simulink model "path_estimation"  (R2023b)
settings: Solver=FixedStepAuto  StartTime=0.0  StopTime=inf  RelTol=1e-3  EnableMultiTasking=on
undefined symbols (not defined in the file): hw
libraries: matrix_library x42, dspadpt3 x20, raspberrypiAVlib x2, audiosources x1
settings Model: ExtModeTrigDuration=2  Creator=mykni  LastModifiedBy=aaron
settings SolverCC: PositivePriorityOrder=on
settings OptimizationCC: EnhancedBackFolding=on  PassReuseOutputArgsAs=Individual arguments  ZeroExternalMemoryAtStartup=off  ZeroInternalMemoryAtStartup=off  MaxStackSize=64  OptimizeBlockOrder=speed  DifferentSizesBufferReuse=on  OptimizationCustomize=off  EfficientTunableParamExpr=on
settings DebuggingCC: ParameterTunabilityLossMsg=error
settings HardwareCC: ProdBitPerPointer=32  ProdBitPerSizeT=32  ProdBitPerPtrDiffT=32  ProdLargestAtomicInteger=Long  ProdLargestAtomicFloat=Double  ProdWordSize=32  ProdLongLongMode=on  ProdHWDeviceType=ARM Compatible->ARM Cortex  UseEmbeddedCoderFeatures=off  UseSimulinkCoderFeatures=off
settings RTWCC: Description=Embedded Coder  SystemTargetFile=ert.tlc  HardwareBoard=Raspberry Pi  TLCOptions="-aInlineSetEventsForThisBaseRateFcn=TLC_FALSE -aSuppressMultiTaskScheduler=TLC_FALSE  -aRateBasedStepFcn=0"  TemplateMakefile=ert_default_tmf  Toolchain=GNU GCC Embedded Linux  BuildConfiguration=Faster Runs
settings CodeAppCC: ForceParamTrailComments=on  IgnoreCustomStorageClasses=off  OperatorAnnotations=on  SimulinkDataObjDesc=on  SFDataObjDesc=on  InsertBlockDesc=on
settings ERTTargetCC: SupportNonInlinedSFcns=on  SupportVariableSizeSignals=on  ExtModeTransport=2  ExtModeStaticAlloc=on  ExtModeMexFile=ext_xcp  ExtModeIntrfLevel=Level2 - Open

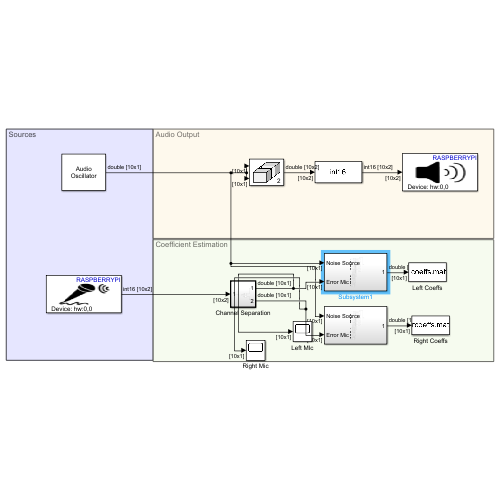
[thumbnail: Simulink's stored preview of the top-level diagram]
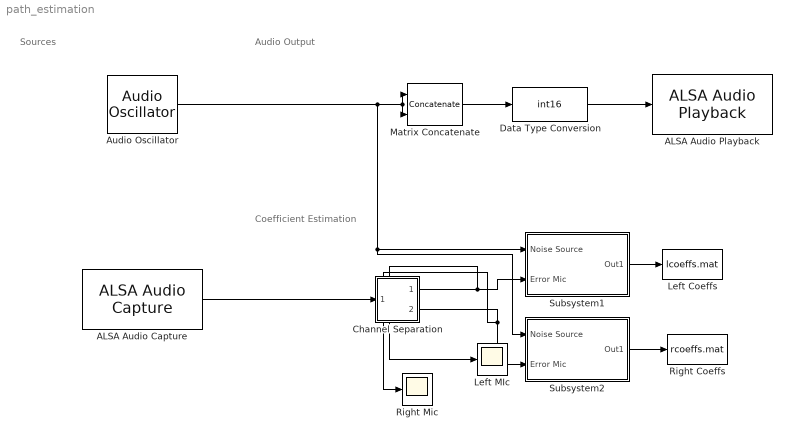
== system path_estimation ==
  note: Audio Output
  note: Coefficient Estimation
  note: Sources
  ALSA Audio Capture : raspberrypiAVlib/ALSA Audio Capture  deviceStr=hw:0,0  DataBitDepth=16-bit integer  numberOfChannels=2  sampleRateEnum=44100  frameSize=10  QueueDuration=0.5  blockPlatform=LINUX
  ALSA Audio Playback : raspberrypiAVlib/ALSA Audio Playback  deviceStr=hw:0,0  sampleRateEnum=44100  queueDuration=0.5  blockPlatform=LINUX
  Audio Oscillator : audiosources/Audio Oscillator  FrequencyPort=off  Frequency=300  AmplitudePort=off  Amplitude=3*10^4  DCOffsetPort=off  PhaseOffset=0  DCOffset=0  WidthPort=off  Width=1  DutyCyclePort=off  DutyCycle=0.5  SampsPerFrame=10  Fs=44100  OutputDataType=double  SimulateUsing=Code generation
      settings: SignalType=sine
  Channel Separation : Subsystem  TreatAsAtomicUnit=on
  Data Type Conversion : DataTypeConversion  OutDataTypeStr=int16  SaturateOnIntegerOverflow=off  RndMeth=Floor
  Left Coeffs : ToFile  Filename=lcoeffs.mat
  Left MIc : Scope
  Matrix Concatenate : Concatenate  Mode=Multidimensional array  ConcatenateDimension=2
  Right Coeffs : ToFile  Filename=rcoeffs.mat
  Right Mic : Scope
  Subsystem1 : Subsystem
  Subsystem2 : Subsystem
  wires:
  Matrix Concatenate/1 -> Data Type Conversion/1
  Audio Oscillator/1 -> Matrix Concatenate/2, Matrix Concatenate/1, Subsystem2/1(Noise Source), Subsystem1/1(Noise Source)
  ALSA Audio Capture/1 -> Channel Separation/1(In1)
  Channel Separation/1(Out1) -> Left MIc/1, Subsystem1/2(Error Mic)
  Channel Separation/2(Out2) -> Right Mic/1, Subsystem2/2(Error Mic)
  Data Type Conversion/1 -> ALSA Audio Playback/1
  Subsystem1/1(Out1) -> Left Coeffs/1
  Subsystem2/1(Out1) -> Right Coeffs/1

== system path_estimation/Channel Separation ==
  In1 : Inport
  Cast To Double : DataTypeConversion  OutDataTypeStr=double  SaturateOnIntegerOverflow=off  RndMeth=Floor
  Submatrix : matrix_library/Submatrix  RowSpan=All rows  RowStartMode=First  RowStartIndex=1  RowEndMode=Last  RowEndIndex=1  ColSpan=One column  ColStartMode=First  ColStartIndex=1  ColEndMode=Last  ColEndIndex=1
  Submatrix1 : matrix_library/Submatrix  RowSpan=All rows  RowStartMode=First  RowStartIndex=1  RowEndMode=Last  RowEndIndex=1  ColSpan=One column  ColStartMode=Last  ColStartIndex=1  ColEndMode=Last  ColEndIndex=1
  Out1 : Outport
  Out2 : Outport  Port=2
  wires:
  Submatrix1/1 -> Out2/1
  Submatrix/1 -> Out1/1
  Cast To Double/1 -> Submatrix1/1, Submatrix/1
  In1/1 -> Cast To Double/1

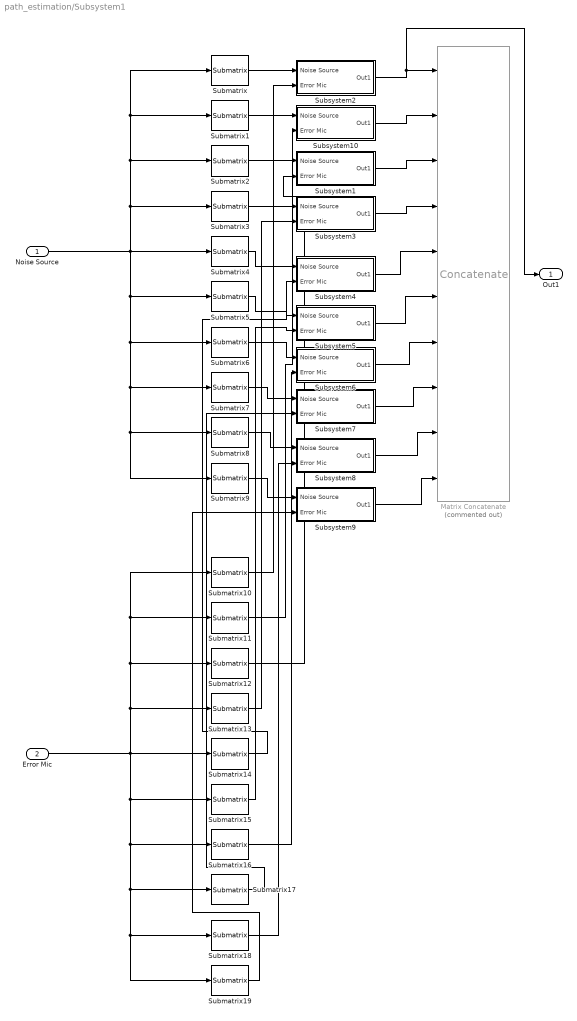
== system path_estimation/Subsystem1 ==
  Noise Source : Inport
  Error Mic : Inport  Port=2
  Matrix Concatenate : Concatenate  Commented=on  NumInputs=10  Mode=Multidimensional array
  Submatrix : matrix_library/Submatrix  RowSpan=One row  RowStartMode=Index  RowStartIndex=1  RowEndMode=Last  RowEndIndex=1  ColSpan=One column  ColStartMode=First  ColStartIndex=1  ColEndMode=Last  ColEndIndex=1
  Submatrix1 : matrix_library/Submatrix  RowSpan=One row  RowStartMode=Index  RowStartIndex=2  RowEndMode=Last  RowEndIndex=1  ColSpan=One column  ColStartMode=First  ColStartIndex=1  ColEndMode=Last  ColEndIndex=1
  Submatrix10 : matrix_library/Submatrix  RowSpan=One row  RowStartMode=Index  RowStartIndex=1  RowEndMode=Last  RowEndIndex=1  ColSpan=One column  ColStartMode=First  ColStartIndex=1  ColEndMode=Last  ColEndIndex=1
  Submatrix11 : matrix_library/Submatrix  RowSpan=One row  RowStartMode=Index  RowStartIndex=2  RowEndMode=Last  RowEndIndex=1  ColSpan=One column  ColStartMode=First  ColStartIndex=1  ColEndMode=Last  ColEndIndex=1
  Submatrix12 : matrix_library/Submatrix  RowSpan=One row  RowStartMode=Index  RowStartIndex=3  RowEndMode=Last  RowEndIndex=1  ColSpan=One column  ColStartMode=First  ColStartIndex=1  ColEndMode=Last  ColEndIndex=1
  Submatrix13 : matrix_library/Submatrix  RowSpan=One row  RowStartMode=Index  RowStartIndex=4  RowEndMode=Last  RowEndIndex=1  ColSpan=One column  ColStartMode=First  ColStartIndex=1  ColEndMode=Last  ColEndIndex=1
  Submatrix14 : matrix_library/Submatrix  RowSpan=One row  RowStartMode=Index  RowStartIndex=5  RowEndMode=Last  RowEndIndex=1  ColSpan=One column  ColStartMode=First  ColStartIndex=1  ColEndMode=Last  ColEndIndex=1
  Submatrix15 : matrix_library/Submatrix  RowSpan=One row  RowStartMode=Index  RowStartIndex=6  RowEndMode=Last  RowEndIndex=1  ColSpan=One column  ColStartMode=First  ColStartIndex=1  ColEndMode=Last  ColEndIndex=1
  Submatrix16 : matrix_library/Submatrix  RowSpan=One row  RowStartMode=Index  RowStartIndex=7  RowEndMode=Last  RowEndIndex=1  ColSpan=One column  ColStartMode=First  ColStartIndex=1  ColEndMode=Last  ColEndIndex=1
  Submatrix17 : matrix_library/Submatrix  RowSpan=One row  RowStartMode=Index  RowStartIndex=8  RowEndMode=Last  RowEndIndex=1  ColSpan=One column  ColStartMode=First  ColStartIndex=1  ColEndMode=Last  ColEndIndex=1
  Submatrix18 : matrix_library/Submatrix  RowSpan=One row  RowStartMode=Index  RowStartIndex=9  RowEndMode=Last  RowEndIndex=1  ColSpan=One column  ColStartMode=First  ColStartIndex=1  ColEndMode=Last  ColEndIndex=1
  Submatrix19 : matrix_library/Submatrix  RowSpan=One row  RowStartMode=Index  RowStartIndex=10  RowEndMode=Last  RowEndIndex=1  ColSpan=One column  ColStartMode=First  ColStartIndex=1  ColEndMode=Last  ColEndIndex=1
  Submatrix2 : matrix_library/Submatrix  RowSpan=One row  RowStartMode=Index  RowStartIndex=3  RowEndMode=Last  RowEndIndex=1  ColSpan=One column  ColStartMode=First  ColStartIndex=1  ColEndMode=Last  ColEndIndex=1
  Submatrix3 : matrix_library/Submatrix  RowSpan=One row  RowStartMode=Index  RowStartIndex=4  RowEndMode=Last  RowEndIndex=1  ColSpan=One column  ColStartMode=First  ColStartIndex=1  ColEndMode=Last  ColEndIndex=1
  Submatrix4 : matrix_library/Submatrix  RowSpan=One row  RowStartMode=Index  RowStartIndex=5  RowEndMode=Last  RowEndIndex=1  ColSpan=One column  ColStartMode=First  ColStartIndex=1  ColEndMode=Last  ColEndIndex=1
  Submatrix5 : matrix_library/Submatrix  RowSpan=One row  RowStartMode=Index  RowStartIndex=6  RowEndMode=Last  RowEndIndex=1  ColSpan=One column  ColStartMode=First  ColStartIndex=1  ColEndMode=Last  ColEndIndex=1
  Submatrix6 : matrix_library/Submatrix  RowSpan=One row  RowStartMode=Index  RowStartIndex=7  RowEndMode=Last  RowEndIndex=1  ColSpan=One column  ColStartMode=First  ColStartIndex=1  ColEndMode=Last  ColEndIndex=1
  Submatrix7 : matrix_library/Submatrix  RowSpan=One row  RowStartMode=Index  RowStartIndex=8  RowEndMode=Last  RowEndIndex=1  ColSpan=One column  ColStartMode=First  ColStartIndex=1  ColEndMode=Last  ColEndIndex=1
  Submatrix8 : matrix_library/Submatrix  RowSpan=One row  RowStartMode=Index  RowStartIndex=9  RowEndMode=Last  RowEndIndex=1  ColSpan=One column  ColStartMode=First  ColStartIndex=1  ColEndMode=Last  ColEndIndex=1
  Submatrix9 : matrix_library/Submatrix  RowSpan=One row  RowStartMode=Index  RowStartIndex=10  RowEndMode=Last  RowEndIndex=1  ColSpan=One column  ColStartMode=First  ColStartIndex=1  ColEndMode=Last  ColEndIndex=1
  Subsystem1 : Subsystem
  Subsystem10 : Subsystem
  Subsystem2 : Subsystem
  Subsystem3 : Subsystem
  Subsystem4 : Subsystem
  Subsystem5 : Subsystem
  Subsystem6 : Subsystem
  Subsystem7 : Subsystem
  Subsystem8 : Subsystem
  Subsystem9 : Subsystem
  Out1 : Outport
  wires:
  Noise Source/1 -> Submatrix9/1, Submatrix8/1, Submatrix7/1, Submatrix6/1, Submatrix5/1, Submatrix/1, Submatrix1/1, Submatrix2/1, Submatrix3/1, Submatrix4/1
  Submatrix/1 -> Subsystem2/1(Noise Source)
  Error Mic/1 -> Submatrix19/1, Submatrix18/1, Submatrix17/1, Submatrix16/1, Submatrix15/1, Submatrix10/1, Submatrix11/1, Submatrix12/1, Submatrix13/1, Submatrix14/1
  Submatrix10/1 -> Subsystem2/2(Error Mic)
  Submatrix1/1 -> Subsystem10/1(Noise Source)
  Submatrix11/1 -> Subsystem10/2(Error Mic)
  Submatrix2/1 -> Subsystem1/1(Noise Source)
  Submatrix12/1 -> Subsystem1/2(Error Mic)
  Submatrix3/1 -> Subsystem3/1(Noise Source)
  Submatrix13/1 -> Subsystem3/2(Error Mic)
  Submatrix4/1 -> Subsystem4/1(Noise Source)
  Submatrix14/1 -> Subsystem4/2(Error Mic)
  Subsystem4/1(Out1) -> Matrix Concatenate/5
  Submatrix5/1 -> Subsystem5/1(Noise Source)
  Submatrix15/1 -> Subsystem5/2(Error Mic)
  Subsystem5/1(Out1) -> Matrix Concatenate/6
  Submatrix6/1 -> Subsystem6/1(Noise Source)
  Submatrix16/1 -> Subsystem6/2(Error Mic)
  Submatrix17/1 -> Subsystem7/2(Error Mic)
  Submatrix7/1 -> Subsystem7/1(Noise Source)
  Subsystem7/1(Out1) -> Matrix Concatenate/8
  Subsystem6/1(Out1) -> Matrix Concatenate/7
  Subsystem8/1(Out1) -> Matrix Concatenate/9
  Subsystem9/1(Out1) -> Matrix Concatenate/10
  Submatrix8/1 -> Subsystem8/1(Noise Source)
  Submatrix9/1 -> Subsystem9/1(Noise Source)
  Submatrix18/1 -> Subsystem8/2(Error Mic)
  Submatrix19/1 -> Subsystem9/2(Error Mic)
  Subsystem3/1(Out1) -> Matrix Concatenate/4
  Subsystem2/1(Out1) -> Out1/1, Matrix Concatenate/1
  Subsystem10/1(Out1) -> Matrix Concatenate/2
  Subsystem1/1(Out1) -> Matrix Concatenate/3

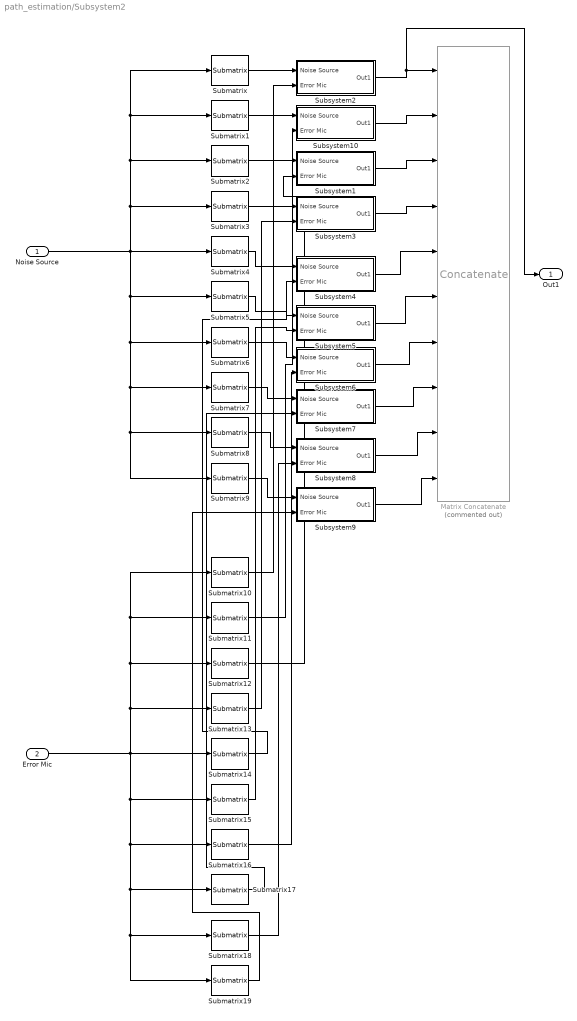
== system path_estimation/Subsystem2 ==
  Noise Source : Inport
  Error Mic : Inport  Port=2
  Matrix Concatenate : Concatenate  Commented=on  NumInputs=10  Mode=Multidimensional array
  Submatrix : matrix_library/Submatrix  RowSpan=One row  RowStartMode=Index  RowStartIndex=1  RowEndMode=Last  RowEndIndex=1  ColSpan=One column  ColStartMode=First  ColStartIndex=1  ColEndMode=Last  ColEndIndex=1
  Submatrix1 : matrix_library/Submatrix  RowSpan=One row  RowStartMode=Index  RowStartIndex=2  RowEndMode=Last  RowEndIndex=1  ColSpan=One column  ColStartMode=First  ColStartIndex=1  ColEndMode=Last  ColEndIndex=1
  Submatrix10 : matrix_library/Submatrix  RowSpan=One row  RowStartMode=Index  RowStartIndex=1  RowEndMode=Last  RowEndIndex=1  ColSpan=One column  ColStartMode=First  ColStartIndex=1  ColEndMode=Last  ColEndIndex=1
  Submatrix11 : matrix_library/Submatrix  RowSpan=One row  RowStartMode=Index  RowStartIndex=2  RowEndMode=Last  RowEndIndex=1  ColSpan=One column  ColStartMode=First  ColStartIndex=1  ColEndMode=Last  ColEndIndex=1
  Submatrix12 : matrix_library/Submatrix  RowSpan=One row  RowStartMode=Index  RowStartIndex=3  RowEndMode=Last  RowEndIndex=1  ColSpan=One column  ColStartMode=First  ColStartIndex=1  ColEndMode=Last  ColEndIndex=1
  Submatrix13 : matrix_library/Submatrix  RowSpan=One row  RowStartMode=Index  RowStartIndex=4  RowEndMode=Last  RowEndIndex=1  ColSpan=One column  ColStartMode=First  ColStartIndex=1  ColEndMode=Last  ColEndIndex=1
  Submatrix14 : matrix_library/Submatrix  RowSpan=One row  RowStartMode=Index  RowStartIndex=5  RowEndMode=Last  RowEndIndex=1  ColSpan=One column  ColStartMode=First  ColStartIndex=1  ColEndMode=Last  ColEndIndex=1
  Submatrix15 : matrix_library/Submatrix  RowSpan=One row  RowStartMode=Index  RowStartIndex=6  RowEndMode=Last  RowEndIndex=1  ColSpan=One column  ColStartMode=First  ColStartIndex=1  ColEndMode=Last  ColEndIndex=1
  Submatrix16 : matrix_library/Submatrix  RowSpan=One row  RowStartMode=Index  RowStartIndex=7  RowEndMode=Last  RowEndIndex=1  ColSpan=One column  ColStartMode=First  ColStartIndex=1  ColEndMode=Last  ColEndIndex=1
  Submatrix17 : matrix_library/Submatrix  RowSpan=One row  RowStartMode=Index  RowStartIndex=8  RowEndMode=Last  RowEndIndex=1  ColSpan=One column  ColStartMode=First  ColStartIndex=1  ColEndMode=Last  ColEndIndex=1
  Submatrix18 : matrix_library/Submatrix  RowSpan=One row  RowStartMode=Index  RowStartIndex=9  RowEndMode=Last  RowEndIndex=1  ColSpan=One column  ColStartMode=First  ColStartIndex=1  ColEndMode=Last  ColEndIndex=1
  Submatrix19 : matrix_library/Submatrix  RowSpan=One row  RowStartMode=Index  RowStartIndex=10  RowEndMode=Last  RowEndIndex=1  ColSpan=One column  ColStartMode=First  ColStartIndex=1  ColEndMode=Last  ColEndIndex=1
  Submatrix2 : matrix_library/Submatrix  RowSpan=One row  RowStartMode=Index  RowStartIndex=3  RowEndMode=Last  RowEndIndex=1  ColSpan=One column  ColStartMode=First  ColStartIndex=1  ColEndMode=Last  ColEndIndex=1
  Submatrix3 : matrix_library/Submatrix  RowSpan=One row  RowStartMode=Index  RowStartIndex=4  RowEndMode=Last  RowEndIndex=1  ColSpan=One column  ColStartMode=First  ColStartIndex=1  ColEndMode=Last  ColEndIndex=1
  Submatrix4 : matrix_library/Submatrix  RowSpan=One row  RowStartMode=Index  RowStartIndex=5  RowEndMode=Last  RowEndIndex=1  ColSpan=One column  ColStartMode=First  ColStartIndex=1  ColEndMode=Last  ColEndIndex=1
  Submatrix5 : matrix_library/Submatrix  RowSpan=One row  RowStartMode=Index  RowStartIndex=6  RowEndMode=Last  RowEndIndex=1  ColSpan=One column  ColStartMode=First  ColStartIndex=1  ColEndMode=Last  ColEndIndex=1
  Submatrix6 : matrix_library/Submatrix  RowSpan=One row  RowStartMode=Index  RowStartIndex=7  RowEndMode=Last  RowEndIndex=1  ColSpan=One column  ColStartMode=First  ColStartIndex=1  ColEndMode=Last  ColEndIndex=1
  Submatrix7 : matrix_library/Submatrix  RowSpan=One row  RowStartMode=Index  RowStartIndex=8  RowEndMode=Last  RowEndIndex=1  ColSpan=One column  ColStartMode=First  ColStartIndex=1  ColEndMode=Last  ColEndIndex=1
  Submatrix8 : matrix_library/Submatrix  RowSpan=One row  RowStartMode=Index  RowStartIndex=9  RowEndMode=Last  RowEndIndex=1  ColSpan=One column  ColStartMode=First  ColStartIndex=1  ColEndMode=Last  ColEndIndex=1
  Submatrix9 : matrix_library/Submatrix  RowSpan=One row  RowStartMode=Index  RowStartIndex=10  RowEndMode=Last  RowEndIndex=1  ColSpan=One column  ColStartMode=First  ColStartIndex=1  ColEndMode=Last  ColEndIndex=1
  Subsystem1 : Subsystem
  Subsystem10 : Subsystem
  Subsystem2 : Subsystem
  Subsystem3 : Subsystem
  Subsystem4 : Subsystem
  Subsystem5 : Subsystem
  Subsystem6 : Subsystem
  Subsystem7 : Subsystem
  Subsystem8 : Subsystem
  Subsystem9 : Subsystem
  Out1 : Outport
  wires:
  Noise Source/1 -> Submatrix9/1, Submatrix8/1, Submatrix7/1, Submatrix6/1, Submatrix5/1, Submatrix/1, Submatrix1/1, Submatrix2/1, Submatrix3/1, Submatrix4/1
  Submatrix/1 -> Subsystem2/1(Noise Source)
  Error Mic/1 -> Submatrix19/1, Submatrix18/1, Submatrix17/1, Submatrix16/1, Submatrix15/1, Submatrix10/1, Submatrix11/1, Submatrix12/1, Submatrix13/1, Submatrix14/1
  Submatrix10/1 -> Subsystem2/2(Error Mic)
  Submatrix1/1 -> Subsystem10/1(Noise Source)
  Submatrix11/1 -> Subsystem10/2(Error Mic)
  Submatrix2/1 -> Subsystem1/1(Noise Source)
  Submatrix12/1 -> Subsystem1/2(Error Mic)
  Submatrix3/1 -> Subsystem3/1(Noise Source)
  Submatrix13/1 -> Subsystem3/2(Error Mic)
  Submatrix4/1 -> Subsystem4/1(Noise Source)
  Submatrix14/1 -> Subsystem4/2(Error Mic)
  Subsystem4/1(Out1) -> Matrix Concatenate/5
  Submatrix5/1 -> Subsystem5/1(Noise Source)
  Submatrix15/1 -> Subsystem5/2(Error Mic)
  Subsystem5/1(Out1) -> Matrix Concatenate/6
  Submatrix6/1 -> Subsystem6/1(Noise Source)
  Submatrix16/1 -> Subsystem6/2(Error Mic)
  Submatrix17/1 -> Subsystem7/2(Error Mic)
  Submatrix7/1 -> Subsystem7/1(Noise Source)
  Subsystem7/1(Out1) -> Matrix Concatenate/8
  Subsystem6/1(Out1) -> Matrix Concatenate/7
  Subsystem8/1(Out1) -> Matrix Concatenate/9
  Subsystem9/1(Out1) -> Matrix Concatenate/10
  Submatrix8/1 -> Subsystem8/1(Noise Source)
  Submatrix9/1 -> Subsystem9/1(Noise Source)
  Submatrix18/1 -> Subsystem8/2(Error Mic)
  Submatrix19/1 -> Subsystem9/2(Error Mic)
  Subsystem3/1(Out1) -> Matrix Concatenate/4
  Subsystem2/1(Out1) -> Out1/1, Matrix Concatenate/1
  Subsystem10/1(Out1) -> Matrix Concatenate/2
  Subsystem1/1(Out1) -> Matrix Concatenate/3

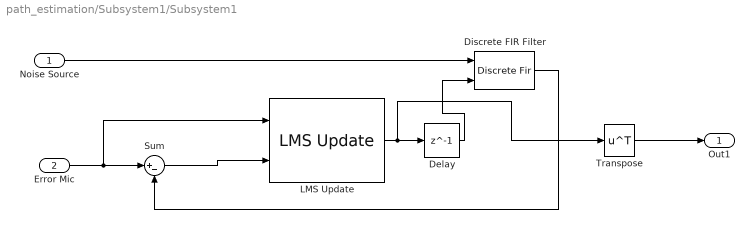
== system path_estimation/Subsystem1/Subsystem1 ==
  Noise Source : Inport
  Error Mic : Inport  Port=2
  Delay : Delay  DelayLength=1  InitialCondition=0
  Discrete FIR Filter : DiscreteFir  CoefSource=Input port
      settings: InputPortMap=u0,u1
  LMS Update : dspadpt3/LMS Update  Method=LMS  Length=10  NumFilters=1  StepSizeSource=Property  StepSize=0.1  LeakageFactor=1.0  InitialConditions=0  AdaptiveFilterMode=Tapped delay-line FIR filter  EnableAdaptInput=off  EnableResetInput=off  SimulateUsing=Code generation
  Sum : Sum  Inputs=|+-
  Transpose : Math  Operator=transpose
  Out1 : Outport
  wires:
  LMS Update/1 -> Transpose/1, Delay/1
  Delay/1 -> Discrete FIR Filter/2
  Noise Source/1 -> Discrete FIR Filter/1
  Error Mic/1 -> LMS Update/1, Sum/1
  Sum/1 -> LMS Update/2
  Discrete FIR Filter/1 -> Sum/2
  Transpose/1 -> Out1/1

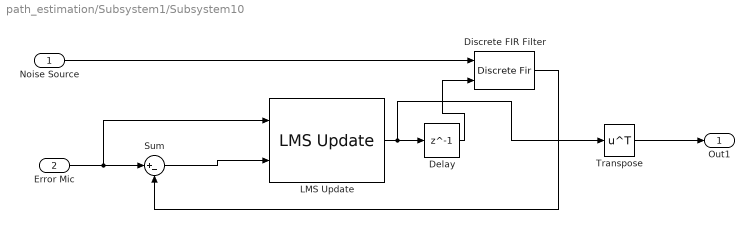
== system path_estimation/Subsystem1/Subsystem10 ==
  Noise Source : Inport
  Error Mic : Inport  Port=2
  Delay : Delay  DelayLength=1  InitialCondition=0
  Discrete FIR Filter : DiscreteFir  CoefSource=Input port
      settings: InputPortMap=u0,u1
  LMS Update : dspadpt3/LMS Update  Method=LMS  Length=10  NumFilters=1  StepSizeSource=Property  StepSize=0.1  LeakageFactor=1.0  InitialConditions=0  AdaptiveFilterMode=Tapped delay-line FIR filter  EnableAdaptInput=off  EnableResetInput=off  SimulateUsing=Code generation
  Sum : Sum  Inputs=|+-
  Transpose : Math  Operator=transpose
  Out1 : Outport
  wires:
  LMS Update/1 -> Transpose/1, Delay/1
  Delay/1 -> Discrete FIR Filter/2
  Noise Source/1 -> Discrete FIR Filter/1
  Error Mic/1 -> LMS Update/1, Sum/1
  Sum/1 -> LMS Update/2
  Discrete FIR Filter/1 -> Sum/2
  Transpose/1 -> Out1/1

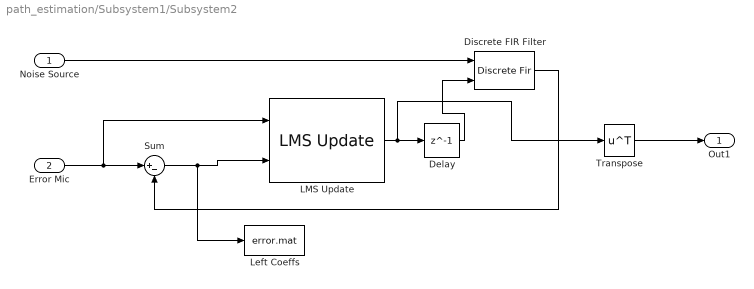
== system path_estimation/Subsystem1/Subsystem2 ==
  Noise Source : Inport
  Error Mic : Inport  Port=2
  Delay : Delay  DelayLength=1  InitialCondition=0
  Discrete FIR Filter : DiscreteFir  CoefSource=Input port
      settings: InputPortMap=u0,u1
  LMS Update : dspadpt3/LMS Update  Method=LMS  Length=10  NumFilters=1  StepSizeSource=Property  StepSize=0.1  LeakageFactor=1.0  InitialConditions=0  AdaptiveFilterMode=Tapped delay-line FIR filter  EnableAdaptInput=off  EnableResetInput=off  SimulateUsing=Code generation
  Left Coeffs : ToFile  Filename=error.mat
  Sum : Sum  Inputs=|+-
  Transpose : Math  Operator=transpose
  Out1 : Outport
  wires:
  LMS Update/1 -> Transpose/1, Delay/1
  Delay/1 -> Discrete FIR Filter/2
  Noise Source/1 -> Discrete FIR Filter/1
  Error Mic/1 -> LMS Update/1, Sum/1
  Sum/1 -> Left Coeffs/1, LMS Update/2
  Discrete FIR Filter/1 -> Sum/2
  Transpose/1 -> Out1/1

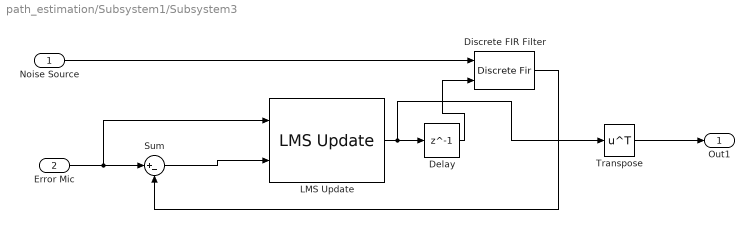
== system path_estimation/Subsystem1/Subsystem3 ==
  Noise Source : Inport
  Error Mic : Inport  Port=2
  Delay : Delay  DelayLength=1  InitialCondition=0
  Discrete FIR Filter : DiscreteFir  CoefSource=Input port
      settings: InputPortMap=u0,u1
  LMS Update : dspadpt3/LMS Update  Method=LMS  Length=10  NumFilters=1  StepSizeSource=Property  StepSize=0.1  LeakageFactor=1.0  InitialConditions=0  AdaptiveFilterMode=Tapped delay-line FIR filter  EnableAdaptInput=off  EnableResetInput=off  SimulateUsing=Code generation
  Sum : Sum  Inputs=|+-
  Transpose : Math  Operator=transpose
  Out1 : Outport
  wires:
  LMS Update/1 -> Transpose/1, Delay/1
  Delay/1 -> Discrete FIR Filter/2
  Noise Source/1 -> Discrete FIR Filter/1
  Error Mic/1 -> LMS Update/1, Sum/1
  Sum/1 -> LMS Update/2
  Discrete FIR Filter/1 -> Sum/2
  Transpose/1 -> Out1/1

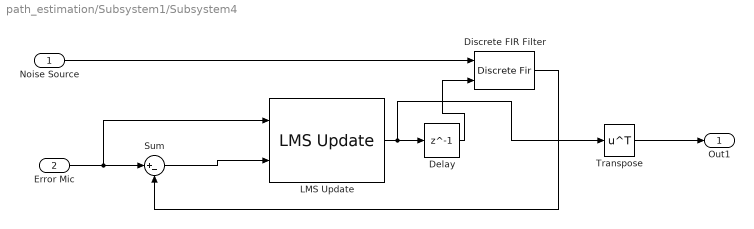
== system path_estimation/Subsystem1/Subsystem4 ==
  Noise Source : Inport
  Error Mic : Inport  Port=2
  Delay : Delay  DelayLength=1  InitialCondition=0
  Discrete FIR Filter : DiscreteFir  CoefSource=Input port
      settings: InputPortMap=u0,u1
  LMS Update : dspadpt3/LMS Update  Method=LMS  Length=10  NumFilters=1  StepSizeSource=Property  StepSize=0.1  LeakageFactor=1.0  InitialConditions=0  AdaptiveFilterMode=Tapped delay-line FIR filter  EnableAdaptInput=off  EnableResetInput=off  SimulateUsing=Code generation
  Sum : Sum  Inputs=|+-
  Transpose : Math  Operator=transpose
  Out1 : Outport
  wires:
  LMS Update/1 -> Transpose/1, Delay/1
  Delay/1 -> Discrete FIR Filter/2
  Noise Source/1 -> Discrete FIR Filter/1
  Error Mic/1 -> LMS Update/1, Sum/1
  Sum/1 -> LMS Update/2
  Discrete FIR Filter/1 -> Sum/2
  Transpose/1 -> Out1/1

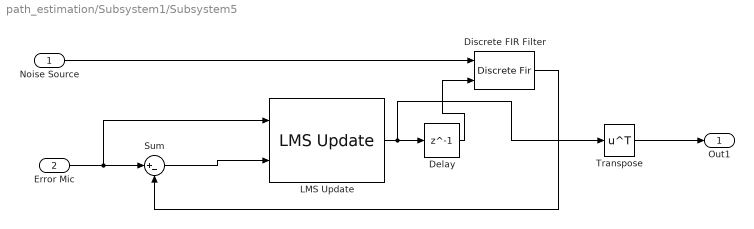
== system path_estimation/Subsystem1/Subsystem5 ==
  Noise Source : Inport
  Error Mic : Inport  Port=2
  Delay : Delay  DelayLength=1  InitialCondition=0
  Discrete FIR Filter : DiscreteFir  CoefSource=Input port
      settings: InputPortMap=u0,u1
  LMS Update : dspadpt3/LMS Update  Method=LMS  Length=10  NumFilters=1  StepSizeSource=Property  StepSize=0.1  LeakageFactor=1.0  InitialConditions=0  AdaptiveFilterMode=Tapped delay-line FIR filter  EnableAdaptInput=off  EnableResetInput=off  SimulateUsing=Code generation
  Sum : Sum  Inputs=|+-
  Transpose : Math  Operator=transpose
  Out1 : Outport
  wires:
  LMS Update/1 -> Transpose/1, Delay/1
  Delay/1 -> Discrete FIR Filter/2
  Noise Source/1 -> Discrete FIR Filter/1
  Error Mic/1 -> LMS Update/1, Sum/1
  Sum/1 -> LMS Update/2
  Discrete FIR Filter/1 -> Sum/2
  Transpose/1 -> Out1/1

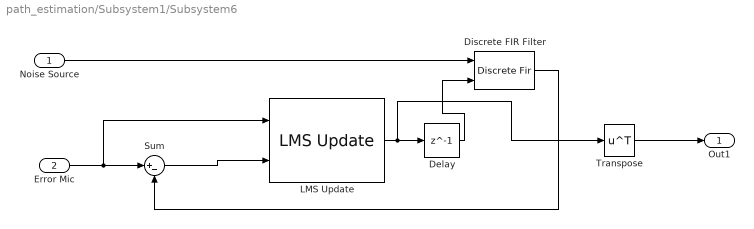
== system path_estimation/Subsystem1/Subsystem6 ==
  Noise Source : Inport
  Error Mic : Inport  Port=2
  Delay : Delay  DelayLength=1  InitialCondition=0
  Discrete FIR Filter : DiscreteFir  CoefSource=Input port
      settings: InputPortMap=u0,u1
  LMS Update : dspadpt3/LMS Update  Method=LMS  Length=10  NumFilters=1  StepSizeSource=Property  StepSize=0.1  LeakageFactor=1.0  InitialConditions=0  AdaptiveFilterMode=Tapped delay-line FIR filter  EnableAdaptInput=off  EnableResetInput=off  SimulateUsing=Code generation
  Sum : Sum  Inputs=|+-
  Transpose : Math  Operator=transpose
  Out1 : Outport
  wires:
  LMS Update/1 -> Transpose/1, Delay/1
  Delay/1 -> Discrete FIR Filter/2
  Noise Source/1 -> Discrete FIR Filter/1
  Error Mic/1 -> LMS Update/1, Sum/1
  Sum/1 -> LMS Update/2
  Discrete FIR Filter/1 -> Sum/2
  Transpose/1 -> Out1/1

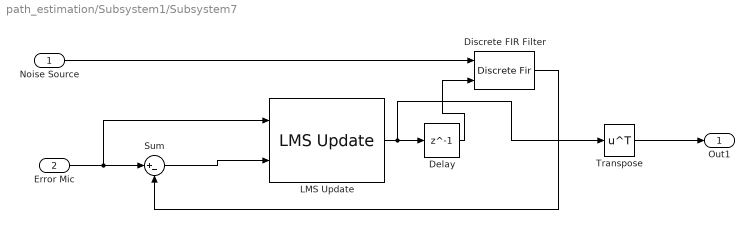
== system path_estimation/Subsystem1/Subsystem7 ==
  Noise Source : Inport
  Error Mic : Inport  Port=2
  Delay : Delay  DelayLength=1  InitialCondition=0
  Discrete FIR Filter : DiscreteFir  CoefSource=Input port
      settings: InputPortMap=u0,u1
  LMS Update : dspadpt3/LMS Update  Method=LMS  Length=10  NumFilters=1  StepSizeSource=Property  StepSize=0.1  LeakageFactor=1.0  InitialConditions=0  AdaptiveFilterMode=Tapped delay-line FIR filter  EnableAdaptInput=off  EnableResetInput=off  SimulateUsing=Code generation
  Sum : Sum  Inputs=|+-
  Transpose : Math  Operator=transpose
  Out1 : Outport
  wires:
  LMS Update/1 -> Transpose/1, Delay/1
  Delay/1 -> Discrete FIR Filter/2
  Noise Source/1 -> Discrete FIR Filter/1
  Error Mic/1 -> LMS Update/1, Sum/1
  Sum/1 -> LMS Update/2
  Discrete FIR Filter/1 -> Sum/2
  Transpose/1 -> Out1/1

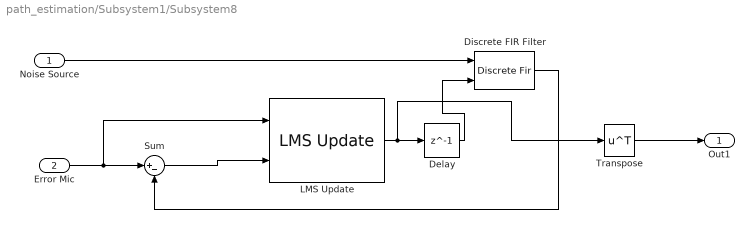
== system path_estimation/Subsystem1/Subsystem8 ==
  Noise Source : Inport
  Error Mic : Inport  Port=2
  Delay : Delay  DelayLength=1  InitialCondition=0
  Discrete FIR Filter : DiscreteFir  CoefSource=Input port
      settings: InputPortMap=u0,u1
  LMS Update : dspadpt3/LMS Update  Method=LMS  Length=10  NumFilters=1  StepSizeSource=Property  StepSize=0.1  LeakageFactor=1.0  InitialConditions=0  AdaptiveFilterMode=Tapped delay-line FIR filter  EnableAdaptInput=off  EnableResetInput=off  SimulateUsing=Code generation
  Sum : Sum  Inputs=|+-
  Transpose : Math  Operator=transpose
  Out1 : Outport
  wires:
  LMS Update/1 -> Transpose/1, Delay/1
  Delay/1 -> Discrete FIR Filter/2
  Noise Source/1 -> Discrete FIR Filter/1
  Error Mic/1 -> LMS Update/1, Sum/1
  Sum/1 -> LMS Update/2
  Discrete FIR Filter/1 -> Sum/2
  Transpose/1 -> Out1/1

== system path_estimation/Subsystem1/Subsystem9 ==
  Noise Source : Inport
  Error Mic : Inport  Port=2
  Delay : Delay  DelayLength=1  InitialCondition=0
  Discrete FIR Filter : DiscreteFir  CoefSource=Input port
      settings: InputPortMap=u0,u1
  LMS Update : dspadpt3/LMS Update  Method=LMS  Length=10  NumFilters=1  StepSizeSource=Property  StepSize=0.1  LeakageFactor=1.0  InitialConditions=0  AdaptiveFilterMode=Tapped delay-line FIR filter  EnableAdaptInput=off  EnableResetInput=off  SimulateUsing=Code generation
  Sum : Sum  Inputs=|+-
  Transpose : Math  Operator=transpose
  Out1 : Outport
  wires:
  LMS Update/1 -> Transpose/1, Delay/1
  Delay/1 -> Discrete FIR Filter/2
  Noise Source/1 -> Discrete FIR Filter/1
  Error Mic/1 -> LMS Update/1, Sum/1
  Sum/1 -> LMS Update/2
  Discrete FIR Filter/1 -> Sum/2
  Transpose/1 -> Out1/1

== system path_estimation/Subsystem2/Subsystem1 ==
  Noise Source : Inport
  Error Mic : Inport  Port=2
  Delay : Delay  DelayLength=1  InitialCondition=0
  Discrete FIR Filter : DiscreteFir  CoefSource=Input port
      settings: InputPortMap=u0,u1
  LMS Update : dspadpt3/LMS Update  Method=LMS  Length=10  NumFilters=1  StepSizeSource=Property  StepSize=0.1  LeakageFactor=1.0  InitialConditions=0  AdaptiveFilterMode=Tapped delay-line FIR filter  EnableAdaptInput=off  EnableResetInput=off  SimulateUsing=Code generation
  Sum : Sum  Inputs=|+-
  Transpose : Math  Operator=transpose
  Out1 : Outport
  wires:
  LMS Update/1 -> Transpose/1, Delay/1
  Delay/1 -> Discrete FIR Filter/2
  Noise Source/1 -> Discrete FIR Filter/1
  Error Mic/1 -> LMS Update/1, Sum/1
  Sum/1 -> LMS Update/2
  Discrete FIR Filter/1 -> Sum/2
  Transpose/1 -> Out1/1

== system path_estimation/Subsystem2/Subsystem10 ==
  Noise Source : Inport
  Error Mic : Inport  Port=2
  Delay : Delay  DelayLength=1  InitialCondition=0
  Discrete FIR Filter : DiscreteFir  CoefSource=Input port
      settings: InputPortMap=u0,u1
  LMS Update : dspadpt3/LMS Update  Method=LMS  Length=10  NumFilters=1  StepSizeSource=Property  StepSize=0.1  LeakageFactor=1.0  InitialConditions=0  AdaptiveFilterMode=Tapped delay-line FIR filter  EnableAdaptInput=off  EnableResetInput=off  SimulateUsing=Code generation
  Sum : Sum  Inputs=|+-
  Transpose : Math  Operator=transpose
  Out1 : Outport
  wires:
  LMS Update/1 -> Transpose/1, Delay/1
  Delay/1 -> Discrete FIR Filter/2
  Noise Source/1 -> Discrete FIR Filter/1
  Error Mic/1 -> LMS Update/1, Sum/1
  Sum/1 -> LMS Update/2
  Discrete FIR Filter/1 -> Sum/2
  Transpose/1 -> Out1/1

== system path_estimation/Subsystem2/Subsystem2 ==
  Noise Source : Inport
  Error Mic : Inport  Port=2
  Delay : Delay  DelayLength=1  InitialCondition=0
  Discrete FIR Filter : DiscreteFir  CoefSource=Input port
      settings: InputPortMap=u0,u1
  LMS Update : dspadpt3/LMS Update  Method=LMS  Length=10  NumFilters=1  StepSizeSource=Property  StepSize=0.1  LeakageFactor=1.0  InitialConditions=0  AdaptiveFilterMode=Tapped delay-line FIR filter  EnableAdaptInput=off  EnableResetInput=off  SimulateUsing=Code generation
  Sum : Sum  Inputs=|+-
  Transpose : Math  Operator=transpose
  Out1 : Outport
  wires:
  LMS Update/1 -> Transpose/1, Delay/1
  Delay/1 -> Discrete FIR Filter/2
  Noise Source/1 -> Discrete FIR Filter/1
  Error Mic/1 -> LMS Update/1, Sum/1
  Sum/1 -> LMS Update/2
  Discrete FIR Filter/1 -> Sum/2
  Transpose/1 -> Out1/1

== system path_estimation/Subsystem2/Subsystem3 ==
  Noise Source : Inport
  Error Mic : Inport  Port=2
  Delay : Delay  DelayLength=1  InitialCondition=0
  Discrete FIR Filter : DiscreteFir  CoefSource=Input port
      settings: InputPortMap=u0,u1
  LMS Update : dspadpt3/LMS Update  Method=LMS  Length=10  NumFilters=1  StepSizeSource=Property  StepSize=0.1  LeakageFactor=1.0  InitialConditions=0  AdaptiveFilterMode=Tapped delay-line FIR filter  EnableAdaptInput=off  EnableResetInput=off  SimulateUsing=Code generation
  Sum : Sum  Inputs=|+-
  Transpose : Math  Operator=transpose
  Out1 : Outport
  wires:
  LMS Update/1 -> Transpose/1, Delay/1
  Delay/1 -> Discrete FIR Filter/2
  Noise Source/1 -> Discrete FIR Filter/1
  Error Mic/1 -> LMS Update/1, Sum/1
  Sum/1 -> LMS Update/2
  Discrete FIR Filter/1 -> Sum/2
  Transpose/1 -> Out1/1

== system path_estimation/Subsystem2/Subsystem4 ==
  Noise Source : Inport
  Error Mic : Inport  Port=2
  Delay : Delay  DelayLength=1  InitialCondition=0
  Discrete FIR Filter : DiscreteFir  CoefSource=Input port
      settings: InputPortMap=u0,u1
  LMS Update : dspadpt3/LMS Update  Method=LMS  Length=10  NumFilters=1  StepSizeSource=Property  StepSize=0.1  LeakageFactor=1.0  InitialConditions=0  AdaptiveFilterMode=Tapped delay-line FIR filter  EnableAdaptInput=off  EnableResetInput=off  SimulateUsing=Code generation
  Sum : Sum  Inputs=|+-
  Transpose : Math  Operator=transpose
  Out1 : Outport
  wires:
  LMS Update/1 -> Transpose/1, Delay/1
  Delay/1 -> Discrete FIR Filter/2
  Noise Source/1 -> Discrete FIR Filter/1
  Error Mic/1 -> LMS Update/1, Sum/1
  Sum/1 -> LMS Update/2
  Discrete FIR Filter/1 -> Sum/2
  Transpose/1 -> Out1/1

== system path_estimation/Subsystem2/Subsystem5 ==
  Noise Source : Inport
  Error Mic : Inport  Port=2
  Delay : Delay  DelayLength=1  InitialCondition=0
  Discrete FIR Filter : DiscreteFir  CoefSource=Input port
      settings: InputPortMap=u0,u1
  LMS Update : dspadpt3/LMS Update  Method=LMS  Length=10  NumFilters=1  StepSizeSource=Property  StepSize=0.1  LeakageFactor=1.0  InitialConditions=0  AdaptiveFilterMode=Tapped delay-line FIR filter  EnableAdaptInput=off  EnableResetInput=off  SimulateUsing=Code generation
  Sum : Sum  Inputs=|+-
  Transpose : Math  Operator=transpose
  Out1 : Outport
  wires:
  LMS Update/1 -> Transpose/1, Delay/1
  Delay/1 -> Discrete FIR Filter/2
  Noise Source/1 -> Discrete FIR Filter/1
  Error Mic/1 -> LMS Update/1, Sum/1
  Sum/1 -> LMS Update/2
  Discrete FIR Filter/1 -> Sum/2
  Transpose/1 -> Out1/1

== system path_estimation/Subsystem2/Subsystem6 ==
  Noise Source : Inport
  Error Mic : Inport  Port=2
  Delay : Delay  DelayLength=1  InitialCondition=0
  Discrete FIR Filter : DiscreteFir  CoefSource=Input port
      settings: InputPortMap=u0,u1
  LMS Update : dspadpt3/LMS Update  Method=LMS  Length=10  NumFilters=1  StepSizeSource=Property  StepSize=0.1  LeakageFactor=1.0  InitialConditions=0  AdaptiveFilterMode=Tapped delay-line FIR filter  EnableAdaptInput=off  EnableResetInput=off  SimulateUsing=Code generation
  Sum : Sum  Inputs=|+-
  Transpose : Math  Operator=transpose
  Out1 : Outport
  wires:
  LMS Update/1 -> Transpose/1, Delay/1
  Delay/1 -> Discrete FIR Filter/2
  Noise Source/1 -> Discrete FIR Filter/1
  Error Mic/1 -> LMS Update/1, Sum/1
  Sum/1 -> LMS Update/2
  Discrete FIR Filter/1 -> Sum/2
  Transpose/1 -> Out1/1

== system path_estimation/Subsystem2/Subsystem7 ==
  Noise Source : Inport
  Error Mic : Inport  Port=2
  Delay : Delay  DelayLength=1  InitialCondition=0
  Discrete FIR Filter : DiscreteFir  CoefSource=Input port
      settings: InputPortMap=u0,u1
  LMS Update : dspadpt3/LMS Update  Method=LMS  Length=10  NumFilters=1  StepSizeSource=Property  StepSize=0.1  LeakageFactor=1.0  InitialConditions=0  AdaptiveFilterMode=Tapped delay-line FIR filter  EnableAdaptInput=off  EnableResetInput=off  SimulateUsing=Code generation
  Sum : Sum  Inputs=|+-
  Transpose : Math  Operator=transpose
  Out1 : Outport
  wires:
  LMS Update/1 -> Transpose/1, Delay/1
  Delay/1 -> Discrete FIR Filter/2
  Noise Source/1 -> Discrete FIR Filter/1
  Error Mic/1 -> LMS Update/1, Sum/1
  Sum/1 -> LMS Update/2
  Discrete FIR Filter/1 -> Sum/2
  Transpose/1 -> Out1/1

== system path_estimation/Subsystem2/Subsystem8 ==
  Noise Source : Inport
  Error Mic : Inport  Port=2
  Delay : Delay  DelayLength=1  InitialCondition=0
  Discrete FIR Filter : DiscreteFir  CoefSource=Input port
      settings: InputPortMap=u0,u1
  LMS Update : dspadpt3/LMS Update  Method=LMS  Length=10  NumFilters=1  StepSizeSource=Property  StepSize=0.1  LeakageFactor=1.0  InitialConditions=0  AdaptiveFilterMode=Tapped delay-line FIR filter  EnableAdaptInput=off  EnableResetInput=off  SimulateUsing=Code generation
  Sum : Sum  Inputs=|+-
  Transpose : Math  Operator=transpose
  Out1 : Outport
  wires:
  LMS Update/1 -> Transpose/1, Delay/1
  Delay/1 -> Discrete FIR Filter/2
  Noise Source/1 -> Discrete FIR Filter/1
  Error Mic/1 -> LMS Update/1, Sum/1
  Sum/1 -> LMS Update/2
  Discrete FIR Filter/1 -> Sum/2
  Transpose/1 -> Out1/1

== system path_estimation/Subsystem2/Subsystem9 ==
  Noise Source : Inport
  Error Mic : Inport  Port=2
  Delay : Delay  DelayLength=1  InitialCondition=0
  Discrete FIR Filter : DiscreteFir  CoefSource=Input port
      settings: InputPortMap=u0,u1
  LMS Update : dspadpt3/LMS Update  Method=LMS  Length=10  NumFilters=1  StepSizeSource=Property  StepSize=0.1  LeakageFactor=1.0  InitialConditions=0  AdaptiveFilterMode=Tapped delay-line FIR filter  EnableAdaptInput=off  EnableResetInput=off  SimulateUsing=Code generation
  Sum : Sum  Inputs=|+-
  Transpose : Math  Operator=transpose
  Out1 : Outport
  wires:
  LMS Update/1 -> Transpose/1, Delay/1
  Delay/1 -> Discrete FIR Filter/2
  Noise Source/1 -> Discrete FIR Filter/1
  Error Mic/1 -> LMS Update/1, Sum/1
  Sum/1 -> LMS Update/2
  Discrete FIR Filter/1 -> Sum/2
  Transpose/1 -> Out1/1
